simulink model "Ctrl_For_HRV_20260625"  (R2024b)
settings: Solver=ode4  StartTime=0.0  StopTime=22  FixedStep=0.02  RelTol=1e-3
InitFcn:
  | Parameter;
undefined symbols (not defined in the file or in its folder): CCI_DUI_AngleRate_Controller, CCI_DUI_FlowAngle_Controller, fhan, h_alpha, h_beta, h_miu, h_p, h_q, h_r, PNG_2026_6_23, r_alpha, r_beta, r_miu, r_p, r_q, r_r, xishu, xishu_D_0, xishu_L_0, xishu_l_0, xishu_m_0, xishu_n_0, xishu_Y_0
libraries: simulink x60
(part 6 of 8)

== matlab function Ctrl_For_HRV_20260625/Vehicle_4/HRV_Model_v4/Aerodynamic Parameter perturbation/MATLAB Function ==
  data: state input; dot_state output; u input
function dot_state  = Shedong_Model(state,u)
    C_L_d = state(1);C_D_d = state(2);C_Y_d = state(3);C_l_d = state(4);C_m_d = state(5);C_n_d = state(6);
    xi_L = state(7);xi_D = state(8);xi_Y = state(9);xi_l = state(10);xi_m = state(11);xi_n = state(12);
    omega_C_L_d = u(1);omega_C_D_d = u(2);omega_C_Y_d = u(3);omega_C_l_d = u(4);omega_C_m_d = u(5);omega_C_n_d = u(6);
    omega_xi_L_d = u(7);omega_xi_D_d = u(8);omega_xi_Y_d = u(9);omega_xi_l_d = u(10);omega_xi_m_d = u(11);omega_xi_n_d = u(12);

    dot_C_L_d = -xi_L*C_L_d+omega_C_L_d;    
    dot_C_D_d = -xi_D*C_D_d+omega_C_D_d;
    dot_C_Y_d = -xi_Y*C_Y_d+omega_C_Y_d;
    dot_C_l_d = -xi_l*C_l_d+omega_C_l_d;
    dot_C_m_d = -xi_m*C_m_d+omega_C_m_d;
    dot_C_n_d = -xi_n*C_n_d+omega_C_n_d;
    dot_xi_L = omega_xi_L_d;
    dot_xi_D = omega_xi_D_d;
    dot_xi_Y = omega_xi_Y_d;
    dot_xi_l = omega_xi_l_d;
    dot_xi_m = omega_xi_m_d;
    dot_xi_n = omega_xi_n_d;
            
    dot_state = [dot_C_L_d,dot_C_D_d,dot_C_Y_d,dot_C_l_d,dot_C_m_d,dot_C_n_d,dot_xi_L,dot_xi_D,dot_xi_Y,dot_xi_l,dot_xi_m,dot_xi_n];
end

== matlab function Ctrl_For_HRV_20260625/Vehicle_3/MATLAB Function3_v3 ==
  data: ny_cmd input; alpha_cmd output; nz_cmd input; miu_cmd output; Q input; H input; Ma input; miu_last input; L output
function [alpha_cmd, miu_cmd, L] = fcn(ny_cmd, nz_cmd, Q, H, Ma, miu_last)                                   
% Convert PN load commands to smooth signed alpha and bank commands.                                         
S = 334.73; m = 63504; earth_r = 6371000; g0 = 9.8060;                                                   
sampleTime = 0.02; overloadRateLimit = 50.0;                                                             
alphaRateLimit = 25.0; bankRateLimit = 90.0; commandTau = 0.10;                                          
g = (earth_r/(earth_r + H))^2*g0;                                                                        
persistent nyState nzState alphaState initialized                                                        
if isempty(initialized)                                                                                  
nyState = ny_cmd; nzState = nz_cmd;                                                                  
alphaState = 0.0; initialized = true;                                                                
end                                                                                                      
nyLimited = rateLimit(ny_cmd, nyState, overloadRateLimit, sampleTime);                                   
nzLimited = rateLimit(nz_cmd, nzState, overloadRateLimit, sampleTime);                                   
blend = sampleTime/(commandTau + sampleTime);                                                            
nyState = nyState + blend*(nyLimited - nyState);                                                         
nzState = nzState + blend*(nzLimited - nzState);                                                         
ny = nyState; nz = nzState;                                                                              
nAbs = hypot(ny, nz);                                                                                    
if nAbs < 1e-6                                                                                           
liftSign = 1.0; miu_raw_rad = miu_last*pi/180;                                                       
elseif ny < 0                                                                                            
liftSign = -1.0; miu_raw_rad = atan2(-nz, -ny);                                                      
else                                                                                                     
liftSign = 1.0; miu_raw_rad = atan2(nz, ny);                                                         
end                                                                                                      
miu_raw_rad = saturate(miu_raw_rad, -45*pi/180, 45*pi/180);                                              
miu_last_rad = miu_last*pi/180;                                                                          
miu_target = miu_last_rad + wrapToPiLocal(miu_raw_rad - miu_last_rad);                                   
miu_limited = miu_last_rad + rateLimit(miu_target - miu_last_rad, 0.0, bankRateLimit*pi/180, sampleTime);
miu_cmd = wrapToPiLocal(miu_limited)*180/pi;                                                             
CL_cmd = liftSign*nAbs*m*g/max(Q*S, 1e-6);                                                               
if Ma > 8                                                                                                
alpha_min = -12;                                                                                     
elseif Ma > 5                                                                                            
alpha_min = -12;                                                                                     
else                                                                                                     
alpha_min = -18;                                                                                     
end                                                                                                      
if Ma > 8                                                                                                
alpha_max = 8;                                                                                       
elseif Ma > 5                                                                                            
alpha_max = 10;                                                                                      
elseif Ma > 3                                                                                            
alpha_max = 12;                                                                                      
else                                                                                                     
alpha_max = 14;                                                                                      
end                                                                                                      
CL_min = CL_of_alpha(alpha_min, Ma); CL_max = CL_of_alpha(alpha_max, Ma);                                
CL_cmd = min(max(CL_cmd, min(CL_min, CL_max)), max(CL_min, CL_max));                                     
alphaRaw = solveAlpha(CL_cmd, alpha_min, alpha_max, Ma);                                                 
if alphaState < alpha_min || alphaState > alpha_max                                                      
alphaState = alphaRaw;                                                                               
end                                                                                                      
alphaLimited = rateLimit(alphaRaw, alphaState, alphaRateLimit, sampleTime);                              
alphaState = alphaState + blend*(alphaLimited - alphaState);                                             
alpha_cmd = saturate(alphaState, alpha_min, alpha_max);                                                  
L = CL_cmd;                                                                                              
end                                                                                                          
function alpha = solveAlpha(CL_cmd, alpha_min, alpha_max, Ma)                                                
alpha = alpha_min; bestErr = abs(CL_of_alpha(alpha_min, Ma) - CL_cmd);                                   
for k = 1:120                                                                                            
a = alpha_min + (alpha_max - alpha_min)*k/120;                                                       
err = abs(CL_of_alpha(a, Ma) - CL_cmd);                                                              
if err < bestErr                                                                                     
bestErr = err; alpha = a;                                                                        
end                                                                                                  
end                                                                                                      
end                                                                                                          
function CL = CL_of_alpha(alpha_deg, Ma)                                                                     
CL = (-8.19e-2) + (4.7e-2)*Ma ...                                                                        
+ (1.86e-2)*alpha_deg - (4.73e-4)*(alpha_deg*Ma) ...                                                 
- (9.19e-3)*Ma^2 - (1.52e-4)*alpha_deg^2 ...                                                         
+ (5.99e-7)*(alpha_deg*Ma)^2 + (7.74e-4)*Ma^3 ...                                                    
+ (4.08e-6)*alpha_deg^3 - (2.93e-5)*Ma^4 + (4.12e-7)*Ma^5;                                           
end                                                                                                          
function y = rateLimit(u, yPrev, rateLimitValue, sampleTime)                                                 
maxStep = rateLimitValue*sampleTime;                                                                     
y = yPrev + min(max(u - yPrev, -maxStep), maxStep);                                                      
end                                                                                                          
function y = saturate(x, lo, hi)                                                                             
y = min(max(x, lo), hi);                                                                                 
end                                                                                                          
function ang = wrapToPiLocal(ang)                                                                            
ang = mod(ang + pi, 2*pi) - pi;                                                                          
end

== matlab function Ctrl_For_HRV_20260625/Vehicle_3/PNG/MATLAB Function ==
  data: V input; v output; theta input; psi input
function v = fcn(V,theta,psi)
dot_X = V*cos(theta)*cos(psi);
dot_Y = V*cos(theta)*sin(psi);
dot_H = V*sin(theta);

v=[dot_X;dot_Y;dot_H];

== matlab function Ctrl_For_HRV_20260625/Vehicle_3/PNG/MATLAB Function1 ==
  data: ny_cmd input; alpha_cmd output; nz_cmd input; miu_cmd output; Q input; H input; Ma input; miu_last input
function [alpha_cmd, miu_cmd] = fcn(ny_cmd, nz_cmd, Q, H, Ma, miu_last)                                                                                                                                     
% Convert overload commands to smooth alpha and bank commands.                                                                                                                                              
S = 334.73; m = 63504; earth_r = 6371000; g0 = 9.8060;                                                                                                                                                      
sampleTime = 0.02; overloadRateLimit = 10.0;                                                                                                                                                                
alphaRateLimit = 10.0; bankRateLimit = 30.0*pi/180; commandTau = 0.25;                                                                                                                                      
g = (earth_r/(earth_r + H))^2*g0;                                                                                                                                                                           
persistent nyState nzState alphaState initialized                                                                                                                                                           
if isempty(initialized)                                                                                                                                                                                     
nyState = ny_cmd; nzState = nz_cmd; alphaState = 0.0; initialized = true;                                                                                                                               
end                                                                                                                                                                                                         
nyLimited = rateLimit(ny_cmd, nyState, overloadRateLimit, sampleTime);                                                                                                                                      
nzLimited = rateLimit(nz_cmd, nzState, overloadRateLimit, sampleTime);                                                                                                                                      
blend = sampleTime/(commandTau + sampleTime);                                                                                                                                                               
nyState = nyState + blend*(nyLimited - nyState);                                                                                                                                                            
nzState = nzState + blend*(nzLimited - nzState);                                                                                                                                                            
ny = nyState; nz = nzState;                                                                                                                                                                                 
nL = hypot(ny, nz);                                                                                                                                                                                         
if nL < 1e-4                                                                                                                                                                                                
miu_raw = miu_last;                                                                                                                                                                                     
else                                                                                                                                                                                                        
miu_raw = atan2(ny, nz);                                                                                                                                                                                
end                                                                                                                                                                                                         
miu_target = miu_last + wrapToPiLocal(miu_raw - miu_last);                                                                                                                                                  
miu_cmd = miu_last + rateLimit(miu_target - miu_last, 0.0, bankRateLimit, sampleTime);                                                                                                                      
miu_cmd = wrapToPiLocal(miu_cmd);                                                                                                                                                                           
alpha_min = -30; alpha_max = 30;                                                                                                                                                                            
CL_min = CL_of_alpha(alpha_min, Ma); CL_max = CL_of_alpha(alpha_max, Ma);                                                                                                                                   
CL_cmd = nL*m*g/max(Q*S, 1e-6);                                                                                                                                                                             
CL_cmd = min(max(CL_cmd, min(CL_min, CL_max)), max(CL_min, CL_max));                                                                                                                                        
alphaRaw = solveAlpha(CL_cmd, alpha_min, alpha_max, Ma);                                                                                                                                                    
if alphaState < alpha_min || alphaState > alpha_max                                                                                                                                                         
alphaState = alphaRaw;                                                                                                                                                                                  
end                                                                                                                                                                                                         
alphaLimited = rateLimit(alphaRaw, alphaState, alphaRateLimit, sampleTime);                                                                                                                                 
alphaState = alphaState + blend*(alphaLimited - alphaState);                                                                                                                                                
alpha_cmd = saturate(alphaState, alpha_min, alpha_max);                                                                                                                                                     
end                                                                                                                                                                                                         
function alpha = solveAlpha(CL_cmd, alpha_min, alpha_max, Ma)                                                                                                                                               
alpha = alpha_min; bestErr = abs(CL_of_alpha(alpha_min, Ma) - CL_cmd);                                                                                                                                  
for k = 1:120                                                                                                                                                                                           
a = alpha_min + (alpha_max - alpha_min)*k/120;                                                                                                                                                      
err = abs(CL_of_alpha(a, Ma) - CL_cmd);                                                                                                                                                             
if err < bestErr                                                                                                                                                                                    
bestErr = err; alpha = a;                                                                                                                                                                       
end                                                                                                                                                                                                 
end                                                                                                                                                                                                     
end                                                                                                                                                                                                         
function CL = CL_of_alpha(alpha_deg, Ma)                                                                                                                                                                    
CL = (-8.19e-2)+(4.7e-2)*Ma+(1.86e-2)*alpha_deg-(4.73e-4)*(alpha_deg*Ma)-(9.19e-3)*Ma^2-(1.52e-4)*alpha_deg^2+(5.99e-7)*(alpha_deg*Ma)^2+(7.74e-4)*Ma^3+(4.08e-6)*alpha_deg^3-(2.93e-5)*Ma^4+(4.12e-7)*Ma^5;
end                                                                                                                                                                                                         
function y = rateLimit(u, yPrev, rateLimitValue, sampleTime)                                                                                                                                                
maxStep = rateLimitValue*sampleTime;                                                                                                                                                                        
y = yPrev + min(max(u - yPrev, -maxStep), maxStep);                                                                                                                                                         
end                                                                                                                                                                                                         
function y = saturate(x, lo, hi)                                                                                                                                                                            
y = min(max(x, lo), hi);                                                                                                                                                                                    
end                                                                                                                                                                                                         
function ang = wrapToPiLocal(ang)                                                                                                                                                                           
ang = mod(ang + pi, 2*pi) - pi;                                                                                                                                                                             
end

== matlab function Ctrl_For_HRV_20260625/Vehicle_3/PNG/MATLAB Function2 ==
  data: V input; f_psi output; theta input; psi input; lat input; H input
function f_psi = earth_rotation(V,theta,psi,lat,H)

earth_r = 6371000;
w_e = 7.292116000000000e-05;
R = earth_r + H;
f_psi = V*cos(theta)*sin(psi)*tan(lat)/R ...
      + 2*w_e*(sin(lat)-cos(lat)*cos(psi)*tan(theta)) ...
      + w_e^2*R*cos(lat)*sin(lat)*sin(psi)/(V*cos(theta));

== matlab function Ctrl_For_HRV_20260625/Cooperative_Fuzzy_Guidance ==
  data: h1 input; ny1 output; h2 input; h3 input; h4 input; h5 input; position_t input; vt input; nz1 output; ny2 output; nz2 output; ny3 output; nz3 output; ny4 output; nz4 output; ny5 output; nz5 output; coop_weight output
function [ny1,nz1,ny2,nz2,ny3,nz3,ny4,nz4,ny5,nz5,coop_weight] = fcn(h1,h2,h3,h4,h5,position_t,vt)
% Fuzzy continuous blend of cooperative guidance and PNG from Zhao et al.
H = [h1(:), h2(:), h3(:), h4(:), h5(:)];
n = 5;
pos = [H(7,:); H(9,:); H(8,:)];
V = max(H(4,:), 1.0);
theta = H(5,:); psi = H(6,:); lat = H(3,:); alt = H(1,:);
vel = zeros(3,n);
for i = 1:n
    vel(:,i) = [V(i)*cos(theta(i))*cos(psi(i)); V(i)*cos(theta(i))*sin(psi(i)); V(i)*sin(theta(i))];
end
target = position_t(:); targetVel = vt(:);
A = ones(n,n) - eye(n);
terminalPngRange = 10000.0;
minRange = 1.0; minSpeed = 1.0;
navigationConstant = 4.0;
maxAcceleration = 20.0*9.806;
consensusGain = 0.35;
thetaDesired = [-45.0 -45.0 -45.0 -45.0 -45.0]*pi/180.0;
psiDesired = [17.0 17.0 17.0 17.0 17.0]*pi/180.0;
thetaTerminalGain = [3.0 3.0 3.0 3.0 3.0];
thetaTerminalSign = [1.0 1.0 1.0 1.0 1.0];
thetaDirectLoadGain = [0.0 0.0 0.0 0.0 0.0];
psiTerminalGain = [0.0 0.0 0.0 0.0 0.0];
zemGain = [1.60 1.60 1.60 1.66 1.40];
psiTerminalSign = [-1.0 1.0 -1.0 -1.0 -1.0];
fovMin = 0.0*pi/180.0; fovMax = 80.0*pi/180.0;
xiMin = -cos(fovMin); xiMax = -cos(fovMax);
if xiMin > xiMax
    tmp = xiMin; xiMin = xiMax; xiMax = tmp;
end
xiCenter = 0.5*(xiMin + xiMax);
xiHalfWidth = 0.5*(xiMax - xiMin);
ranges = zeros(1,n); eta = zeros(1,n); xi = zeros(1,n);
lambda = zeros(3,n); lambdaDot = zeros(3,n);
for i = 1:n
    relPos = target - pos(:,i);
    ranges(i) = max(norm(relPos), minRange);
    lambda(:,i) = relPos/ranges(i);
    speed = max(norm(vel(:,i)), minSpeed);
    vhat = vel(:,i)/speed;
    cosDelta = min(max(vhat'*lambda(:,i), -1.0), 1.0);
    xi(i) = -cosDelta;
    eta(i) = ranges(i)/speed;
    relVel = targetVel - vel(:,i);
    lambdaDot(:,i) = (relVel - lambda(:,i)*(lambda(:,i)'*relVel))/ranges(i);
end
L = diag(sum(A,2)) - A;
eEta = (L*eta(:)).';
eXi = (L*xi(:)).';
cooperativeState = mean(abs(eta - mean(eta))) + 20.0*mean(abs(xi - mean(xi)));
Dbar = mean(ranges);
fuzzy_weight = fuzzyCooperativeWeight(cooperativeState, Dbar, terminalPngRange);
nyCmd = zeros(1,n); nzCmd = zeros(1,n);
coop_weight = fuzzy_weight;
for i = 1:n
    [nyPng,nzPng] = terminalPngLoad(pos(:,i), vel(:,i), target, targetVel, V(i), theta(i), psi(i), lat(i), alt(i), thetaDesired(i), psiDesired(i), thetaTerminalGain(i), thetaTerminalSign(i), thetaDirectLoadGain(i), psiTerminalGain(i), psiTerminalSign(i), zemGain(i));
    xiRef = xiCenter - xiHalfWidth*tanh(consensusGain*(eEta(i) + eXi(i)));
    uHat = -consensusGain*(xi(i) - xiRef);
    aCoop = cooperativeAcceleration(vel(:,i), lambda(:,i), lambdaDot(:,i), uHat, minSpeed);
    aCoop = limitVectorMagnitude(aCoop, maxAcceleration);
    [nyCoop,nzCoop] = accelToLoad(aCoop, V(i), theta(i), psi(i), lat(i), alt(i));
    w = 0.0;
    nyCmd(i) = clamp(w*nyCoop + (1.0-w)*nyPng, -20.0, 20.0);
    nzCmd(i) = clamp(w*nzCoop + (1.0-w)*nzPng, -20.0, 20.0);
end
ny1 = nyCmd(1); nz1 = nzCmd(1);
ny2 = nyCmd(2); nz2 = nzCmd(2);
ny3 = nyCmd(3); nz3 = nzCmd(3);
ny4 = nyCmd(4); nz4 = nzCmd(4);
ny5 = nyCmd(5); nz5 = nzCmd(5);
end
function weight = fuzzyCooperativeWeight(cooperativeState, averageRange, terminalPngRange)
cooperativeScale = 3.0; fuzzyFarRange = 60000.0; sigma = 0.45;
cooInput = 2.0*clamp(cooperativeState/cooperativeScale, 0.0, 1.0) - 1.0;
rangeInput = 2.0*clamp((averageRange - terminalPngRange)/max(fuzzyFarRange - terminalPngRange, eps), 0.0, 1.0) - 1.0;
centers = [-1.0, 0.0, 1.0];
cooMembership = gaussianMembership(cooInput, centers, sigma);
rangeMembership = gaussianMembership(rangeInput, centers, sigma);
ruleLevels = [-1.0 -1.0 -1.0; -1.0 0.0 1.0; -1.0 0.0 1.0];
num = 0.0; den = 0.0;
for k = 1:401
    y = -1.0 + (k-1)*(2.0/400.0);
    aggregated = 0.0;
    for row = 1:3
        for col = 1:3
            activation = min(rangeMembership(row), cooMembership(col));
            consequent = gaussianMembership(y, ruleLevels(row,col), sigma);
            aggregated = max(aggregated, min(activation, consequent));
        end
    end
    num = num + y*aggregated;
    den = den + aggregated;
end
if den <= eps
    fuzzyOutput = -1.0;
else
    fuzzyOutput = num/den;
end
weight = clamp(0.5*(fuzzyOutput + 1.0), 0.0, 1.0);
end
function [ny,nz] = terminalPngLoad(p, v, target, targetVel, V, theta, psi, lat, H, thetaDesired, psiDesired, KterminalTheta, thetaTerminalSign, KdirectTheta, KterminalPsi, psiTerminalSign, Kzem)
rTrue = target - p;
realRange = max(norm(rTrue), 1.0);
aimpoint = target;
rx = aimpoint(1) - p(1); ry = aimpoint(2) - p(2); rh = aimpoint(3) - p(3);
vr = targetVel - v;
range = max(sqrt(rx*rx + ry*ry + rh*rh), 1.0);
closing = max(-(rx*vr(1) + ry*vr(2) + rh*vr(3))/range, 50.0);
qTheta = atan2(rh, hypot(rx, ry));
qPsi = atan2(ry, rx);
rho2 = max(rx*rx + ry*ry, 1.0);
qPsiDot = (rx*vr(2) - ry*vr(1))/rho2;
rhoriz = sqrt(rho2);
rhorizDot = (rx*vr(1) + ry*vr(2))/rhoriz;
qThetaDot = (rhoriz*vr(3) - rh*rhorizDot)/max(rho2 + rh*rh, 1.0);
thetaErr = wrapToPiLocal(qTheta - theta);
psiErr = wrapToPiLocal(qPsi - psi);
tgo = min(max(range/closing, 1.0), 80.0);
Ntheta = 5.2; Npsi = 6.0; Ktheta = 1.0; Kpsi = 1.3;
terminalThetaErr = thetaTerminalSign*wrapToPiLocal(thetaDesired - theta);
terminalPsiErr = psiTerminalSign*wrapToPiLocal(psiDesired - psi);
terminalBlend = smoothStep((realRange - 25000.0)/(3000.0 - 25000.0));
losBlend = 1.0 - terminalBlend;
aThetaPng = Ntheta*closing*qThetaDot + losBlend*Ktheta*V*thetaErr/tgo + terminalBlend*KterminalTheta*V*terminalThetaErr/tgo;
aPsiPng = Npsi*closing*qPsiDot + losBlend*Kpsi*V*cos(theta)*psiErr/tgo + terminalBlend*KterminalPsi*V*cos(theta)*terminalPsiErr/tgo;
relVelTrue = targetVel - v;
tgoZem = min(max(realRange/max(closing, 50.0), 0.35), 30.0);
zem = rTrue + relVelTrue*tgoZem;
zemBlend = smoothStep((realRange - 9000.0)/(800.0 - 9000.0));
eThetaZem = [-sin(theta)*cos(psi); -sin(theta)*sin(psi); cos(theta)];
ePsiZem = [-sin(psi); cos(psi); 0.0];
zemTheta = zem'*eThetaZem;
zemPsi = zem'*ePsiZem;
aThetaZem = clamp(Kzem*zemTheta/(tgoZem*tgoZem), -2.5*9.806, 2.5*9.806)*zemBlend;
aPsiZem = clamp(Kzem*zemPsi/(tgoZem*tgoZem), -2.5*9.806, 2.5*9.806)*zemBlend;
aTheta = aThetaPng + aThetaZem;
aPsi = aPsiPng + aPsiZem;
earth_r = 6371000.0; omega = 7.292116e-5; g0 = 9.806; R = earth_r + H; g = (earth_r/R)^2*g0;
geomTheta = V*cos(theta)/R + 2.0*omega*cos(lat)*sin(psi) + omega^2*R*cos(lat)*(cos(theta)*cos(lat)+sin(theta)*cos(psi)*sin(lat))/V;
geomPsi = V*cos(theta)*sin(psi)*tan(lat)/R + 2.0*omega*(sin(lat)-cos(lat)*cos(psi)*tan(theta)) + omega^2*R*cos(lat)*sin(lat)*sin(psi)/max(V*cos(theta),1.0);
nyRaw = aTheta/g + cos(theta) - (V/g)*geomTheta + KdirectTheta*terminalBlend*terminalThetaErr;
nz = clamp(aPsi/g - (V*cos(theta)/g)*geomPsi, -20.0, 20.0);
ny = clamp(nyRaw - 0.35*abs(nz), -20.0, 20.0);
end
function aCoop = cooperativeAcceleration(vM, lambda, lambdaDot, uHat, minSpeed)
speed = norm(vM);
if speed < minSpeed
    aCoop = [0.0; 0.0; 0.0];
    return;
end
vhat = vM/speed;
lambdaPerp = lambda - (vhat'*lambda)*vhat;
den = lambdaPerp'*lambdaPerp;
if den < 1.0e-8
    aCoop = [0.0; 0.0; 0.0];
    return;
end
rhs = -speed*(uHat + vhat'*lambdaDot);
aCoop = rhs*lambdaPerp/den;
aCoop = removeAxialComponent(aCoop, vM, minSpeed);
end
function [ny,nz] = accelToLoad(a, V, theta, psi, lat, H)
earth_r = 6371000.0; omega = 7.292116e-5; g0 = 9.806; R = earth_r + H;
g = (earth_r/R)^2*g0;
eTheta = [-sin(theta)*cos(psi); -sin(theta)*sin(psi); cos(theta)];
ePsi = [-sin(psi); cos(psi); 0.0];
aTheta = a'*eTheta;
aPsi = a'*ePsi;
geomTheta = V*cos(theta)/R + 2.0*omega*cos(lat)*sin(psi) + omega^2*R*cos(lat)*(cos(theta)*cos(lat)+sin(theta)*cos(psi)*sin(lat))/V;
geomPsi = V*cos(theta)*sin(psi)*tan(lat)/R + 2.0*omega*(sin(lat)-cos(lat)*cos(psi)*tan(theta)) + omega^2*R*cos(lat)*sin(lat)*sin(psi)/max(V*cos(theta),1.0);
ny = clamp(aTheta/g + cos(theta) - (V/g)*geomTheta, -20.0, 20.0);
nz = clamp(aPsi/g - (V*cos(theta)/g)*geomPsi, -20.0, 20.0);
end
function a = removeAxialComponent(a, v, minSpeed)
speed = norm(v);
if speed < minSpeed
    return;
end
vhat = v/speed;
a = a - (a'*vhat)*vhat;
end
function y = limitVectorMagnitude(x, maxMagnitude)
xNorm = norm(x);
if xNorm > maxMagnitude && xNorm > 0.0
    y = x*(maxMagnitude/xNorm);
else
    y = x;
end
end
function y = gaussianMembership(x, centers, sigma)
y = exp(-((x - centers).^2)/(2.0*sigma*sigma));
end
function y = smoothStep(x)
x = clamp(x, 0.0, 1.0);
y = x*x*(3.0 - 2.0*x);
end
function angle = wrapToPiLocal(angle)
angle = mod(angle + pi, 2.0*pi) - pi;
end
function y = clamp(x, lo, hi)
y = min(max(x, lo), hi);
end

== matlab function Ctrl_For_HRV_20260625/Vehicle_4/Hit_Detection_v4 ==
  settings: updateMethod=DISCRETE  sampleTime=0.02
  data: r_mt output; position_t input; stop output; hgv_states input
function [r_mt,stop] = fcn(position_t, hgv_states)
% Stop simulation once the continuous segment crosses the hit radius.
hitRadius = 10;
p = [hgv_states(7); hgv_states(9); hgv_states(8)];
t = [position_t(1); position_t(2); position_t(3)];
persistent prevP initialized
if isempty(initialized)
    prevP = p;
    initialized = true;
end
d = p - t;
pointDist2 = d(1)*d(1) + d(2)*d(2) + d(3)*d(3);
seg = p - prevP;
den = seg(1)*seg(1) + seg(2)*seg(2) + seg(3)*seg(3);
if den > 0.0
    u = ((t(1)-prevP(1))*seg(1) + (t(2)-prevP(2))*seg(2) + (t(3)-prevP(3))*seg(3))/den;
    u = min(max(u, 0.0), 1.0);
else
    u = 1.0;
end
closest = prevP + u*seg;
e = closest - t;
segDist2 = e(1)*e(1) + e(2)*e(2) + e(3)*e(3);
stop = segDist2 <= hitRadius*hitRadius;
r_mt = sqrt(pointDist2);
prevP = p;
end

== matlab function Ctrl_For_HRV_20260625/Vehicle_4/MATLAB Function_v4 ==
  settings: updateMethod=DISCRETE
  data: alpha input; alpha_noise output; beta input; miu input; p input; q input; r input; beta_noise output; miu_noise output; p_noise output; q_noise output; r_noise output
function [alpha_noise,beta_noise,miu_noise,p_noise,q_noise,r_noise]= fcn(alpha,beta,miu,p,q,r)

% alpha_noise = awgn(alpha,100);
% beta_noise = awgn(beta,100);
% miu_noise = awgn(miu,100);
% p_noise = awgn(p,100);
% q_noise = awgn(q,100);
% r_noise = awgn(r,100);

alpha_noise = alpha;
beta_noise = beta;
miu_noise = miu;
p_noise = p;
q_noise = q;
r_noise = r;

== matlab function Ctrl_For_HRV_20260625/Vehicle_4/MATLAB Function1 ==
  data: u input; y output
function y = fcn(u)

omega_c = [alpha_c;beta_c;miu_c];
dot_omega_c = [dot_alpha_c;dot_beta_c;dot_miu_c];
ddot_omega_c = [ddot_alpha_c;ddot_beta_c;ddot_miu_c];
e_wd = [e_wd_1;e_wd_2;e_wd_3];
dot_e_wd = [dot_e_wd_1;dot_e_wd_2;dot_e_wd_3];

[Ma,Q] = M_Q(H,V);
%计算气动系数
[C_L_alpha,C_L_delta_a,C_L_delta_e] = Coefficient_Lift(alpha,Ma,delta_a,delta_e,delta_r);
[C_D_alpha,C_D_delta_a,C_D_delta_e,C_D_delta_r] = Coefficient_Drag(alpha,Ma,delta_a,delta_e,delta_r);
[C_Y_beta,C_Y_delta_a,C_Y_delta_e,C_Y_delta_r] = Coefficient_Side(alpha,Ma,delta_a,delta_e,delta_r);
% [C_L_alpha,C_L_delta_a,C_L_delta_e] = Coefficient_Lift(alpha,Ma,0,0,0);
% [C_D_alpha,C_D_delta_a,C_D_delta_e,C_D_delta_r] = Coefficient_Drag(alpha,Ma,0,0,0);
% [C_Y_beta,C_Y_delta_a,C_Y_delta_e,C_Y_delta_r] = Coefficient_Side(alpha,Ma,0,0,0);
[C_l_beta,C_l_delta_a,C_l_delta_e,C_l_delta_r,C_l_r,C_l_p] = Coefficient_RollingMoment(alpha,Ma,delta_a,delta_e,delta_r);
[C_m_alpha,C_m_delta_a,C_m_delta_e,C_m_delta_r,C_m_q] = Coefficient_PitchMoment(alpha,Ma,delta_a,delta_e,delta_r);
[C_n_beta,C_n_delta_a,C_n_delta_e,C_n_delta_r,C_n_p,C_n_r] = Coefficient_YawingMoment(alpha,Ma,delta_a,delta_e,delta_r);
C_L = C_L_alpha+C_L_delta_a+C_L_delta_e;
C_D = C_D_alpha+C_D_delta_a+C_D_delta_e+C_D_delta_r;
C_Y = C_Y_beta*beta+C_Y_delta_a+C_Y_delta_e+C_Y_delta_r;
C_l = C_l_beta*beta+C_l_delta_a*delta_a+C_l_delta_e*delta_e+C_l_delta_r*delta_r+C_l_r*(r*b/(2*V))+C_l_p*(p*b/(2*V));
C_m = C_m_alpha+C_m_delta_a*delta_a+C_m_delta_e*delta_e+C_m_delta_r*delta_r+C_m_q*(q*c/(2*V));
C_n = C_n_beta*beta+C_n_delta_a*delta_a+C_n_delta_e*delta_e+C_n_delta_r*delta_r+C_n_p*(p*b/(2*V))+C_n_r*(r*b/(2*V));

%摄动值
Delta_C_L = C_L_d*C_L; Delta_C_D = C_D_d*C_D; Delta_C_Y = C_Y_d*C_Y;
Delta_C_l = C_l_d*C_l; Delta_C_m = C_m_d*C_m; Delta_C_n = C_n_d*C_n;

%%重力加速度
R = earth_r+H; %R为地心距
g = (earth_r/R)^2*g0;

%%
% 模型调整
%先得到系数
Coefficient_C_L_alpha = 1.86e-2 + 1.01e-4 + 1.01e-4;
C_L_else = C_L - Coefficient_C_L_alpha * alpha;

Coefficient_C_Y_alpha = -1.12e-7 + 1.12e-7 + 4.86e-20;
C_Y_else = C_Y - Coefficient_C_Y_alpha * alpha;

Coefficient_C_l_beta_0 = -1.402e-1;
C_l_beta_else = C_l_beta - Coefficient_C_l_beta_0;

Coefficient_C_l_p_0 = -2.99e-1;
C_l_p_else = C_l_p - Coefficient_C_l_p_0;

Coefficient_C_l_r_0 = 3.82e-1;
C_l_r_else = C_l_r - Coefficient_C_l_r_0;

Coefficient_C_m_alpha_alpha = -2.260e-3 -6.59e-5 -6.59e-5;
C_m_alpha_else = C_m_alpha - Coefficient_C_m_alpha_alpha*alpha;

Coefficient_C_m_q_0 = -1.36;
C_m_q_else = C_m_q - Coefficient_C_m_q_0;

Coefficient_C_n_p_0 = 3.68e-1;
C_n_p_else = C_n_p - Coefficient_C_n_p_0;


%将模改写为面向控制的形式
d_alpha = 0.1*0.005*sin(0.2*pi*t); d_beta = 0.1*0.005*sin(0.2*pi*t); d_miu = 0.1*0.005*sin(0.2*pi*t);
d_p = 0.1*0.007*sin(pi*t); d_q = 0.1*0.01*sin(pi*t); d_r = 0;
%姿态角环
omega = [alpha;beta;miu];
w = [p;q;r];
u = [delta_a;delta_e;delta_r];

W_oo = [-Q*S*Coefficient_C_L_alpha,0,0;
        Q*S*Coefficient_C_Y_alpha,0,0;
        Q*S*(Coefficient_C_L_alpha*(tan(theta)*sin(miu)+tan(beta))+Coefficient_C_Y_alpha*tan(theta)*cos(beta)*cos(miu))];
F_else = [-Q*S*C_L_else,0,0;
        Q*S*C_Y_else,0,0;
        Q*S*(C_L_else*(tan(theta)*sin(miu)+tan(beta))+C_Y_else*tan(theta)*cos(beta)*cos(miu))];
f_o = [(m*g*cos(theta)*cos(miu))/(m*V*cos(beta));
       (m*g*cos(theta)*sin(miu))/(m*V);
       (-m*g*cos(theta)*tan(beta)*cos(miu))/(m*V)];
g_o = [-p*cos(alpha)*tan(beta) - r*sin(alpha)*tan(beta);
       p*sin(alpha);
       r*sin(alpha)*sec(beta)];
W_ow = [0,1,0;
        0,0,-cos(alpha);
        cos(alpha)*sec(beta)];
phi_s = [(-Q*S*Delta_C_L)/(m*V*cos(beta))+d_alpha;
         (Q*S*Delta_C_Y)/(m*V)+d_beta;
         (Q*S*Delta_C_L*(tan(theta)*sin(miu)+tan(beta))+Q*S*Delta_C_Y*tan(theta)*cos(beta)*cos(miu))/(m*V)+d_miu];
D_F = f_o + F_else + phi_s;
Dot_o = W_oo*omega + W_ow*w + g_o + D_F;

%角速度环
W_wo = [0,Q*S*b*Coefficient_C_l_beta_0/I_xx,0;
        Q*S*c_A*Coefficient_C_m_alpha_alpha/I_yy,0,0;
        0,0,0];
W_ww = [(Q*S*b/I_xx)*(Coefficient_C_l_p_0*b/(2*V)),0,(Q*S*b/I_xx)*(Coefficient_C_l_r_0*b/(2*V));
        0,(Q*S*c_A/I_yy)*Coefficient_C_m_q_0*c_A/(2*V),0;
        (Q*S*b/I_zz)*Coefficient_C_n_p_0*b/(2*V),0,0];
M_else = [(Q*S*b/I_xx)*(C_l_beta_else*beta+C_l_p_else*(p*b/(2*V))+C_l_r_else*(r*b/(2*V)));
          (Q*S*c_A/I_yy)*(C_m_alpha_else+C_m_q_else*(q*c_A/(2*V)));
          (Q*S*b/I_zz)*(C_n_beta*beta+C_n_p_else*(p*b/(2*V))+C_n_r*(r*b/(2*V)))];
f_w = [(I_yy-I_zz)*q*r/I_xx;
       (I_zz-I_xx)*p*r/I_yy;
       (I_xx-I_yy)*p*q/I_zz];
g_f = [Q*S*b*C_l_delta_a/I_xx   Q*S*b*C_l_delta_e/I_xx   Q*S*b*C_l_delta_r/I_xx;
       Q*S*c_A*C_m_delta_a/I_yy Q*S*c_A*C_m_delta_e/I_yy Q*S*c_A*C_m_delta_r/I_yy;
       Q*S*b*C_n_delta_a/I_zz   Q*S*b*C_n_delta_e/I_zz   Q*S*b*C_n_delta_r/I_zz];
phi_f = [Q*S*b*Delta_C_l/I_xx+d_p;
         Q*S*c_A*Delta_C_m/I_yy+d_q;
         Q*S*b*Delta_C_n/I_zz+d_r];
D_M = M_else + phi_f;

Dot_w = W_ww*w + W_wo*omega + g_f*u + f_w + D_M;
%%
%计算误差系统
%e_omega = omega - omega_c;
%e_w = W_ow*w + W_oo*omega_c - dot_omega_c - e_wd;

A_oo = W_oo;
A_ww = W_ow*W_ww*inv(W_ow);
A_wo = W_ow*W_wo;
B = W_ow*g_f;
h = (W_ow*W_wo - W_ow*W_ww*inv(W_ow)*W_oo)*omega_c + (W_oo+W_ow*W_ww*inv(W_ow))*dot_omega_c - ddot_omega_c;
r = W_ow*W_ww*inv(W_ow)*e_wd - dot_e_wd;
D_M_error = W_ow*D_M;

dot_e_omega = A_oo*e_omega + e_w + e_wd + g_o + D_F;
dot_e_w = A_ww*e_w + A_wo*e_omega + f_w + B*u + h + r + D_M_error;


dot_error_alpha = dot_e_omega(1); dot_error_beta = dot_e_omega(2); dot_error_miu = dot_e_omega(3);
dot_error_w_1 = dot_e_w(1); dot_error_w_2 = dot_e_w(2); dot_error_w_3 = dot_e_w(3);

x_dot=[dot_error_alpha;dot_error_beta;dot_error_miu;dot_error_w_1;dot_error_w_2;dot_error_w_3];
sys = x_dot;



y = u;

== matlab function Ctrl_For_HRV_20260625/Vehicle_5/HRV_Model_v5/Aerodynamic Parameter perturbation/MATLAB Function ==
  data: state input; dot_state output; u input
function dot_state  = Shedong_Model(state,u)
    C_L_d = state(1);C_D_d = state(2);C_Y_d = state(3);C_l_d = state(4);C_m_d = state(5);C_n_d = state(6);
    xi_L = state(7);xi_D = state(8);xi_Y = state(9);xi_l = state(10);xi_m = state(11);xi_n = state(12);
    omega_C_L_d = u(1);omega_C_D_d = u(2);omega_C_Y_d = u(3);omega_C_l_d = u(4);omega_C_m_d = u(5);omega_C_n_d = u(6);
    omega_xi_L_d = u(7);omega_xi_D_d = u(8);omega_xi_Y_d = u(9);omega_xi_l_d = u(10);omega_xi_m_d = u(11);omega_xi_n_d = u(12);

    dot_C_L_d = -xi_L*C_L_d+omega_C_L_d;    
    dot_C_D_d = -xi_D*C_D_d+omega_C_D_d;
    dot_C_Y_d = -xi_Y*C_Y_d+omega_C_Y_d;
    dot_C_l_d = -xi_l*C_l_d+omega_C_l_d;
    dot_C_m_d = -xi_m*C_m_d+omega_C_m_d;
    dot_C_n_d = -xi_n*C_n_d+omega_C_n_d;
    dot_xi_L = omega_xi_L_d;
    dot_xi_D = omega_xi_D_d;
    dot_xi_Y = omega_xi_Y_d;
    dot_xi_l = omega_xi_l_d;
    dot_xi_m = omega_xi_m_d;
    dot_xi_n = omega_xi_n_d;
            
    dot_state = [dot_C_L_d,dot_C_D_d,dot_C_Y_d,dot_C_l_d,dot_C_m_d,dot_C_n_d,dot_xi_L,dot_xi_D,dot_xi_Y,dot_xi_l,dot_xi_m,dot_xi_n];
end
